simulink model "Golf_Nonlin_Classique"  (R2019a)
settings: Solver=VariableStepAuto  StartTime=0.0  StopTime=7  RelTol=1e-3
values from neighbouring files (symbols this model uses):
  dPHRTrim = trimVal(1)    [mainProjetCADV_2a.m]
  dthrIdle = 0.1    [mainProjetCADV_2a.m]
  km = trim.kmass(choix)    [utGetTrimPoint.m]
  ms = trim.mStat(choix)    [utGetTrimPoint.m]
  RAD2DEG = 180/pi    (= 57.2957795131)    [mainProjetCADV_2a.m]    (also in utAcDynamicsFunction.m)
  thetaTrim = trimVal(3)    [mainProjetCADV_2a.m]
  uTrim = zeros(TOTAL_CMD, 1)    [mainProjetCADV_2a.m]
  xTrim = zeros(TOTAL_SV, 1)    [mainProjetCADV_2a.m]
undefined symbols (not defined in the file or in its folder): aircraftChosen, Kd, Ki, Kp
settings Model: Creator=bourdiul  LastModifiedBy=ulyss

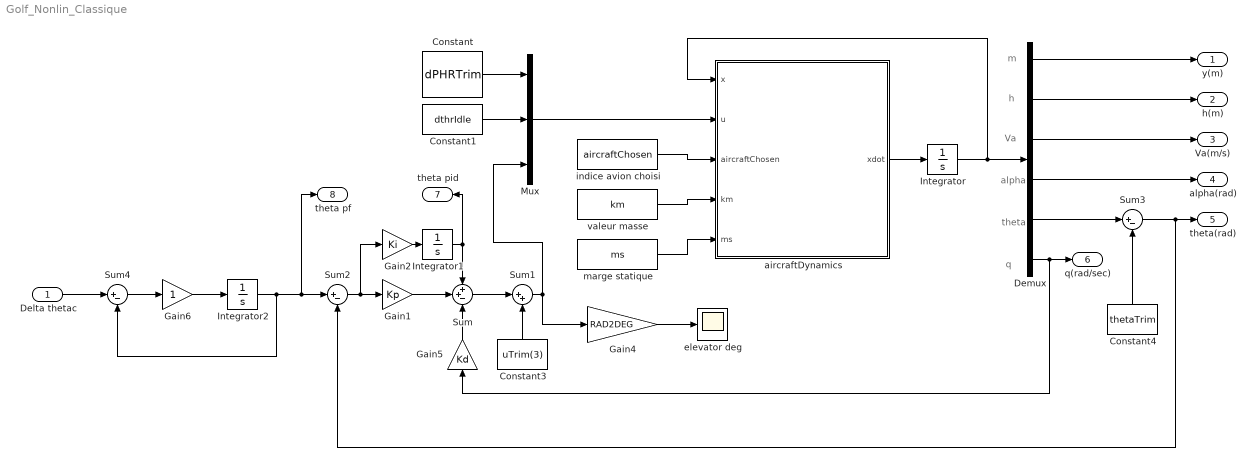
== system Golf_Nonlin_Classique ==
  note: m
  note: h
  note: Va
  note: alpha
  note: theta
  note: q
  "Delta thetac " : Inport
  Constant : Constant  Value=dPHRTrim
  Constant1 : Constant  Value=dthrIdle
  Constant3 : Constant  Value=uTrim(3)
  Constant4 : Constant  Value=thetaTrim
  Demux : Demux  Outputs=6
  Gain1 : Gain  Gain=Kp
  Gain2 : Gain  Gain=Ki
  Gain4 : Gain  Gain=RAD2DEG
  Gain5 : Gain  Gain=Kd
  Gain6 : Gain
  Integrator : Integrator  InitialCondition=xTrim
  Integrator1 : Integrator
  Integrator2 : Integrator
  Mux : Mux  Inputs=3
  Sum : Sum  Inputs=++-
  Sum1 : Sum  Inputs=|++
  Sum2 : Sum  Inputs=|+-
  Sum3 : Sum  Inputs=|+-
  Sum4 : Sum  Inputs=|+-
  aircraftDynamics : MATLAB Function  TreatAsAtomicUnit=on
  elevator deg : Scope
  indice avion choisi : Constant  Value=aircraftChosen
  marge statique : Constant  Value=ms
  valeur masse : Constant  Value=km
  y(m) : Outport
  h(m) : Outport  Port=2
  Va(m/s) : Outport  Port=3
  alpha(rad) : Outport  Port=4
  theta(rad) : Outport  Port=5
  q(rad/sec) : Outport  Port=6
  theta pid : Outport  Port=7
  "theta pf " : Outport  Port=8
  wires:
  marge statique/1 -> aircraftDynamics/5(ms)
  Integrator/1 -> Demux/1, aircraftDynamics/1(x)
  Demux/6 -> Gain5/1, q(rad/sec)/1
  Mux/1 -> aircraftDynamics/2(u)
  Demux/2 -> h(m)/1
  indice avion choisi/1 -> aircraftDynamics/3(aircraftChosen)
  Demux/3 -> Va(m/s)/1
  valeur masse/1 -> aircraftDynamics/4(km)
  aircraftDynamics/1(xdot) -> Integrator/1
  Demux/4 -> alpha(rad)/1
  Constant1/1 -> Mux/2
  Constant/1 -> Mux/1
  Demux/1 -> y(m)/1
  Gain5/1 -> Sum/3
  Gain4/1 -> elevator deg/1
  Constant4/1 -> Sum3/2
  Gain1/1 -> Sum/2
  Integrator1/1 -> theta pid/1, Sum/1
  Gain2/1 -> Integrator1/1
  Sum2/1 -> Gain2/1, Gain1/1
  Demux/5 -> Sum3/1
  Sum3/1 -> theta(rad)/1, Sum2/2
  Integrator2/1 -> "theta pf "/1, Sum2/1, Sum4/2
  Gain6/1 -> Integrator2/1
  Sum4/1 -> Gain6/1
  Constant3/1 -> Sum1/2
  Sum/1 -> Sum1/1
  Sum1/1 -> Gain4/1, Mux/3
  "Delta thetac "/1 -> Sum4/1

== matlab function Golf_Nonlin_Classique/aircraftDynamics ==
  data: x input; u input; xdot output; aircraftChosen input; km input; ms input
function xdot = aircraftDynamics(x,u, aircraftChosen,km,ms)
    TOTAL_SV = 6;
    xIn = zeros(TOTAL_SV,1);
    xIn = x;
    
	TOTAL_CMD = 3;
    uIn = zeros(TOTAL_CMD,1);
    uIn = u;
    
    xdot = utAcDynamicsFunction(xIn,uIn, aircraftChosen,km,ms);
end %aircraftDynamics
